simulink model "liu"  (R2024b)
settings: Solver=VariableStepAuto  StartTime=0.0  StopTime=10.0  RelTol=1e-3
settings Model: Creator=DT User  LastModifiedBy=DT User

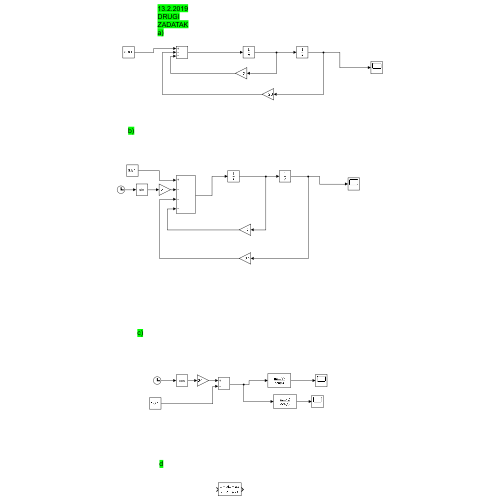
[thumbnail: Simulink's stored preview of the top-level diagram]
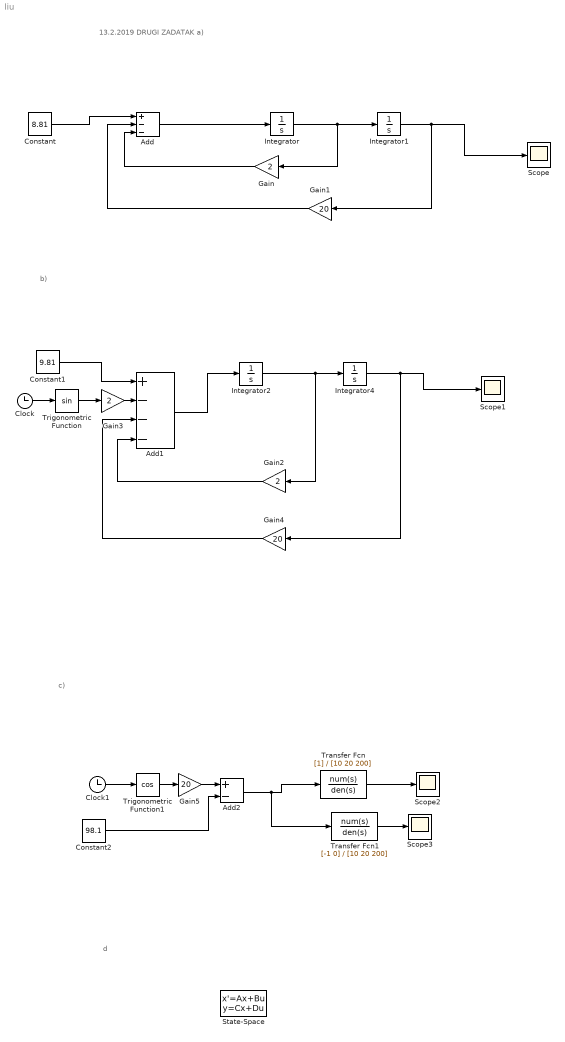
== system liu ==
  note: d
  note: c)
  note: b)
  note: 13.2.2019
      | DRUGI ZADATAK
      | a)
  Add : Sum  Inputs=+--
  Add1 : Sum  Inputs=+---
  Add2 : Sum  Inputs=+-
  Clock : Clock
  Clock1 : Clock
  Constant : Constant  Value=8.81
  Constant1 : Constant  Value=9.81
  Constant2 : Constant  Value=98.1
  Gain : Gain  Gain=2
  Gain1 : Gain  Gain=20
  Gain2 : Gain  Gain=2
  Gain3 : Gain  Gain=2
  Gain4 : Gain  Gain=20
  Gain5 : Gain  Gain=20
  Integrator{,1..2,4} (4 alike) : Integrator
  Scope{,1..3} (4 alike) : Scope
  State-Space : StateSpace  InitialCondition=0
  Transfer Fcn : TransferFcn  Denominator=[10 20 200]
  Transfer Fcn1 : TransferFcn  Numerator=[-1 0]  Denominator=[10 20 200]
  Trigonometric Function : Trigonometry
  Trigonometric Function1 : Trigonometry  Operator=cos
  wires:
  Integrator/1 -> Gain/1, Integrator1/1
  Add/1 -> Integrator/1
  Integrator1/1 -> Gain1/1, Scope/1
  Constant/1 -> Add/1
  Gain/1 -> Add/3
  Gain1/1 -> Add/2
  Integrator2/1 -> Gain2/1, Integrator4/1
  Integrator4/1 -> Gain4/1, Scope1/1
  Clock/1 -> Trigonometric Function/1
  Trigonometric Function/1 -> Gain3/1
  Gain3/1 -> Add1/2
  Constant1/1 -> Add1/1
  Gain2/1 -> Add1/4
  Gain4/1 -> Add1/3
  Add1/1 -> Integrator2/1
  Clock1/1 -> Trigonometric Function1/1
  Trigonometric Function1/1 -> Gain5/1
  Transfer Fcn/1 -> Scope2/1
  Gain5/1 -> Add2/1
  Constant2/1 -> Add2/2
  Add2/1 -> Transfer Fcn1/1, Transfer Fcn/1
  Transfer Fcn1/1 -> Scope3/1
